simulink model "simulink_general_structure_control101"  (R2024a)
settings: Solver=VariableStepAuto  StartTime=0.0  StopTime=endtime  RelTol=1e-3
libraries: cstblocks x3
settings Model: Creator=barsr  LastModifiedBy=Anthony Rossiter
settings RTWCC: GPUComputeCapability=3.5

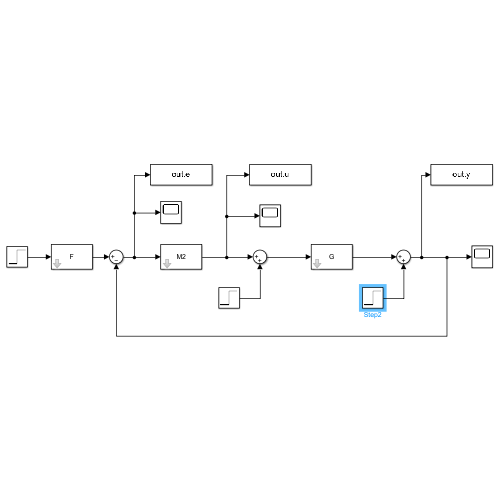
[thumbnail: Simulink's stored preview of the top-level diagram]
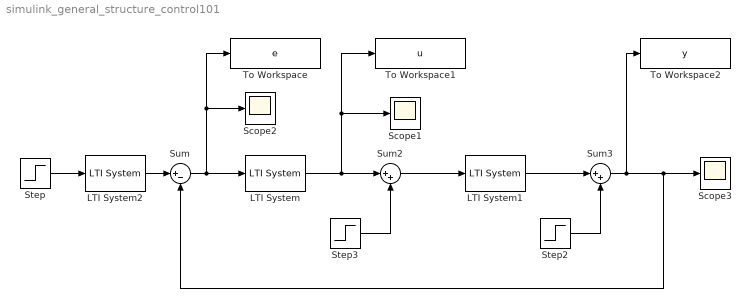
== system simulink_general_structure_control101 ==
  LTI System : cstblocks/LTI System  sys=M2  IC=[]  PadeOrder=0
  LTI System1 : cstblocks/LTI System  sys=G  IC=[]  PadeOrder=0
  LTI System2 : cstblocks/LTI System  sys=F  IC=[]  PadeOrder=0
  Scope1 : Scope
  Scope2 : Scope
  Scope3 : Scope
  Step : Step  Time=0  SampleTime=0
  Step2 : Step  Time=20  After=0.5  SampleTime=0
  Step3 : Step  Time=10  After=0.5  SampleTime=0
  Sum : Sum  Inputs=|+-
  Sum2 : Sum  Inputs=|++
  Sum3 : Sum  Inputs=|++
  To Workspace : ToWorkspace  VariableName=e  SaveFormat=Structure With Time  SampleTime=-1
  To Workspace1 : ToWorkspace  VariableName=u  SaveFormat=Structure With Time  SampleTime=-1
  To Workspace2 : ToWorkspace  VariableName=y  SaveFormat=Structure With Time  SampleTime=-1
  wires:
  Step/1 -> LTI System2/1
  LTI System/1 -> Sum2/1, To Workspace1/1, Scope1/1
  LTI System2/1 -> Sum/1
  Sum2/1 -> LTI System1/1
  LTI System1/1 -> Sum3/1
  Sum/1 -> To Workspace/1, Scope2/1, LTI System/1
  Sum3/1 -> To Workspace2/1, Scope3/1, Sum/2
  Step3/1 -> Sum2/2
  Step2/1 -> Sum3/2
